simulink model "example_code_generation"  (R2024b)
settings: Solver=FixedStepDiscrete  StartTime=0.0  StopTime=40  FixedStep=0.01  RelTol=1e-3
undefined symbols (not defined in the file or in its folder): DiscIntNeverNeededParam
libraries: simulink x19, myLib x19, simulink_extras x8, mcbcontrolslib x2
settings Model: Creator=sakee  LastModifiedBy=sakee

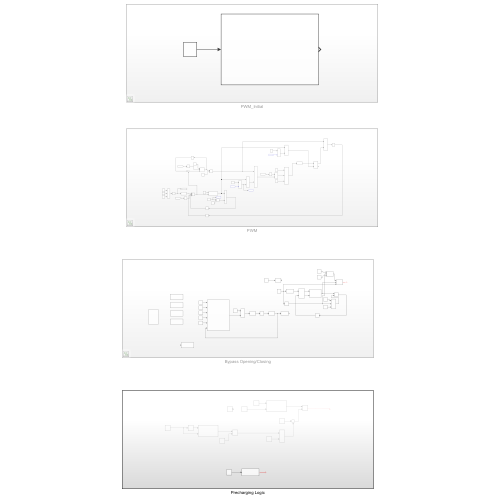
[thumbnail: Simulink's stored preview of the top-level diagram]
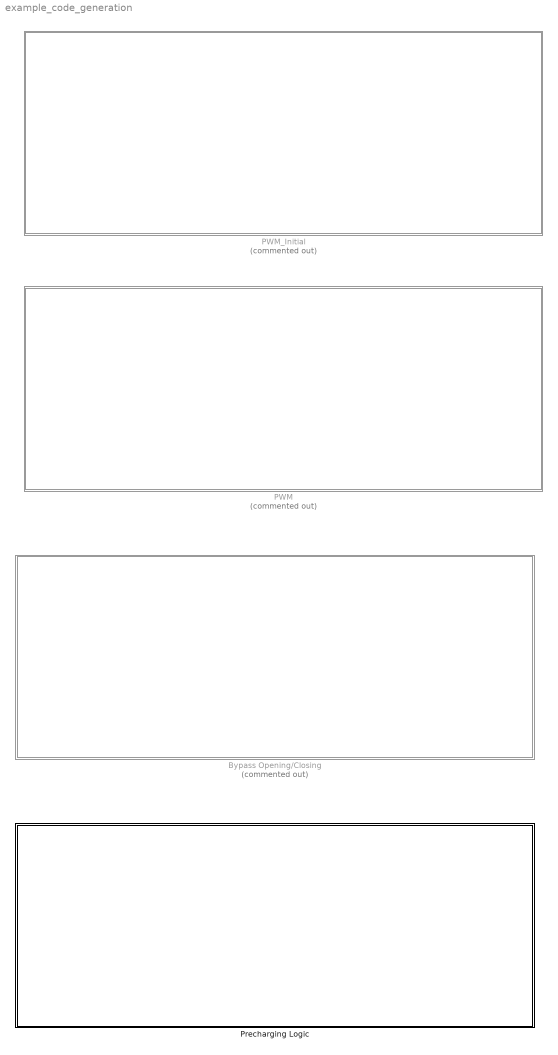
== system example_code_generation ==
  Bypass Opening/Closing : Subsystem  Commented=on
  PWM : Subsystem  Commented=on
  PWM_Initial : Subsystem  Commented=on
  Precharging Logic : Subsystem

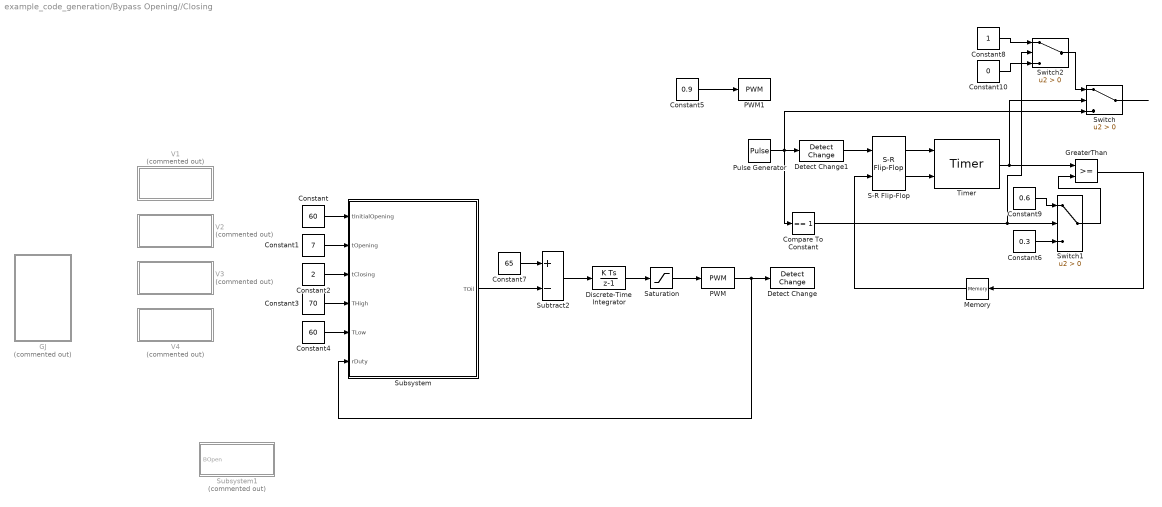
== system example_code_generation/Bypass Opening//Closing ==
  Compare To Constant : simulink/Logic and Bit Operations/Compare To Constant  relop===  const=1  OutDataTypeStr=boolean
  Constant : Constant  Value=60
  Constant1 : Constant  Value=7
  Constant10 : Constant  Value=0
  Constant2 : Constant  Value=2
  Constant3 : Constant  Value=70
  Constant4 : Constant  Value=60
  Constant5 : Constant  Value=0.9
  Constant6 : Constant  Value=0.3
  Constant7 : Constant  Value=65
  Constant8 : Constant
  Constant9 : Constant  Value=0.6
  Detect Change : simulink/Logic and Bit Operations/Detect Change  vinit=0  OutDataTypeStr=boolean
  Detect Change1 : simulink/Logic and Bit Operations/Detect Change  vinit=0  OutDataTypeStr=boolean
  Discrete-Time Integrator : DiscreteIntegrator  gainval=0.05  SampleTime=-1  LimitOutput=on  UpperSaturationLimit=1  LowerSaturationLimit=0  ICPrevOutput=DiscIntNeverNeededParam  ICPrevScaledInput=DiscIntNeverNeededParam
  GJ : Subsystem  Commented=on
  GreaterThan : RelationalOperator  OutDataTypeStr=boolean  RndMeth=Simplest  InputSameDT=off
  Memory : Memory
  PWM : simulink/Discontinuities/PWM  DisableCoverage=on  Period=0.2  InitialDelay=0  DisallowZeroDutyCycle=off  RunAtFixedTimeIntervals=on  SampleTime=0.01
  PWM1 : simulink/Discontinuities/PWM  DisableCoverage=on  Period=0.2  InitialDelay=0  DisallowZeroDutyCycle=off  RunAtFixedTimeIntervals=on  SampleTime=0.01
  Pulse Generator : DiscretePulseGenerator  PulseType=Time based  Period=1  PulseWidth=80
  S-R Flip-Flop : simulink_extras/Flip Flops/S-R Flip-Flop  initial_condition=0
  Saturation : Saturate  UpperLimit=1  LowerLimit=0
  Subsystem : Subsystem
  Subsystem1 : Subsystem  Commented=on
  Subtract2 : Sum  Inputs=+-
  Switch : Switch  Criteria=u2 > Threshold  SaturateOnIntegerOverflow=off  InputSameDT=off
  Switch1 : Switch  Criteria=u2 > Threshold  SaturateOnIntegerOverflow=off  InputSameDT=off
  Switch2 : Switch  Criteria=u2 > Threshold  SaturateOnIntegerOverflow=off  InputSameDT=off
  Timer : myLib/Timer  tSampleTime=0.01
  V1 : Subsystem  Commented=on
  V2 : Subsystem  Commented=on
  V3 : Subsystem  Commented=on
  V4 : Subsystem  Commented=on
  wires:
  Constant/1 -> Subsystem/1(tInitialOpening)
  Constant1/1 -> Subsystem/2(tOpening)
  Constant2/1 -> Subsystem/3(tClosing)
  Constant3/1 -> Subsystem/4(THigh)
  Constant4/1 -> Subsystem/5(TLow)
  Constant7/1 -> Subtract2/1
  Discrete-Time Integrator/1 -> Saturation/1
  Saturation/1 -> PWM/1
  Subtract2/1 -> Discrete-Time Integrator/1
  Subsystem/1(TOil) -> Subtract2/2
  PWM/1 -> Detect Change/1, Subsystem/6(rDuty)
  Constant5/1 -> PWM1/1
  Detect Change1/1 -> S-R Flip-Flop/1
  S-R Flip-Flop/1 -> Timer/1
  S-R Flip-Flop/2 -> Timer/2
  Timer/1 -> Switch/2, GreaterThan/1
  GreaterThan/1 -> Memory/1
  Switch1/1 -> GreaterThan/2
  Memory/1 -> S-R Flip-Flop/2
  Pulse Generator/1 -> Detect Change1/1, Switch/3, Compare To Constant/1
  Switch/1 -> ?
  Compare To Constant/1 -> Switch2/2, Switch1/2
  Constant6/1 -> Switch1/3
  Constant9/1 -> Switch1/1
  Constant8/1 -> Switch2/1
  Constant10/1 -> Switch2/3
  Switch2/1 -> Switch/1

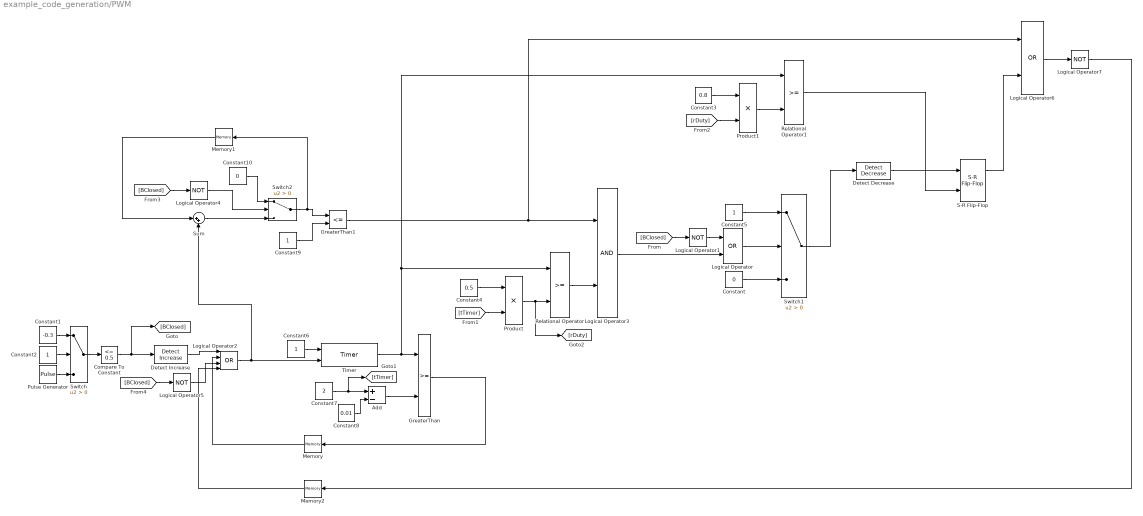
== system example_code_generation/PWM ==
  Add : Sum  Inputs=+-
  Compare To Constant : simulink/Logic and Bit Operations/Compare To Constant  relop=<=  const=0.5  OutDataTypeStr=boolean
  Constant : Constant  Value=0
  Constant1 : Constant  Value=-0.3
  Constant10 : Constant  Value=0
  Constant{2,5..6,9} (4 alike) : Constant
  Constant3 : Constant  Value=0.8
  Constant4 : Constant  Value=0.5
  Constant7 : Constant  Value=2
  Constant8 : Constant  Value=0.01
  Detect Decrease : simulink/Logic and Bit Operations/Detect Decrease  vinit=0.0  OutDataTypeStr=boolean
  Detect Increase : simulink/Logic and Bit Operations/Detect Increase  vinit=0.0  OutDataTypeStr=boolean
  GreaterThan : RelationalOperator  OutDataTypeStr=boolean  RndMeth=Simplest  InputSameDT=off
  GreaterThan1 : RelationalOperator  Operator=<=  OutDataTypeStr=boolean  RndMeth=Simplest  InputSameDT=off
  Logical Operator : Logic  Operator=OR  AllPortsSameDT=off  OutDataTypeStr=boolean
  Logical Operator{1,4..5,7} (4 alike) : Logic  Operator=NOT  AllPortsSameDT=off  OutDataTypeStr=boolean
  Logical Operator2 : Logic  Operator=OR  Inputs=4  AllPortsSameDT=off  OutDataTypeStr=boolean
  Logical Operator3 : Logic  AllPortsSameDT=off  OutDataTypeStr=boolean
  Logical Operator6 : Logic  Operator=OR  AllPortsSameDT=off  OutDataTypeStr=boolean
  Memory : Memory
  Memory1 : Memory
  Memory2 : Memory
  Product : Product
  Product1 : Product
  Pulse Generator : DiscretePulseGenerator  PulseType=Time based  Period=10  PulseWidth=50
  Relational Operator : RelationalOperator  OutDataTypeStr=boolean  RndMeth=Simplest  InputSameDT=off
  Relational Operator1 : RelationalOperator  OutDataTypeStr=boolean  RndMeth=Simplest  InputSameDT=off
  S-R Flip-Flop : simulink_extras/Flip Flops/S-R Flip-Flop  initial_condition=0
  Sum : Sum  Inputs=|++
  Switch : Switch  Criteria=u2 > Threshold  SaturateOnIntegerOverflow=off  InputSameDT=off
  Switch1 : Switch  Criteria=u2 > Threshold  SaturateOnIntegerOverflow=off  InputSameDT=off
  Switch2 : Switch  Criteria=u2 > Threshold  SaturateOnIntegerOverflow=off  InputSameDT=off
  Timer : myLib/Timer  tSampleTime=0.01
  wires:
  Product/1 -> [rDuty], Relational Operator/2
  Compare To Constant/1 -> Detect Increase/1, [BClosed]
  [BClosed] -> Logical Operator1/1
  Constant4/1 -> Product/1
  Constant/1 -> Switch1/3
  Logical Operator/1 -> Switch1/2
  Constant5/1 -> Switch1/1
  Logical Operator1/1 -> Logical Operator/1
  Constant6/1 -> Timer/1
  Pulse Generator/1 -> Switch/3
  Constant2/1 -> Switch/2
  Constant1/1 -> Switch/1
  Switch/1 -> Compare To Constant/1
  Detect Increase/1 -> Logical Operator2/1
  Constant7/1 -> [tTimer], Add/1
  Add/1 -> GreaterThan/2
  Constant8/1 -> Add/2
  GreaterThan/1 -> Memory/1
  Memory/1 -> Logical Operator2/2
  [tTimer] -> Product/2
  Logical Operator3/1 -> Logical Operator/2
  Logical Operator2/1 -> Timer/2, Sum/2
  Constant9/1 -> GreaterThan1/2
  GreaterThan1/1 -> Logical Operator6/1, Logical Operator3/1
  Switch2/1 -> Memory1/1, GreaterThan1/1
  Constant10/1 -> Switch2/1
  Sum/1 -> Switch2/3
  [BClosed] -> Logical Operator4/1
  Logical Operator4/1 -> Switch2/2
  Memory1/1 -> Sum/1
  [BClosed] -> Logical Operator5/1
  Logical Operator5/1 -> Logical Operator2/3
  Relational Operator/1 -> Logical Operator3/2
  Timer/1 -> Relational Operator1/1, Relational Operator/1, GreaterThan/1
  Constant3/1 -> Product1/1
  Product1/1 -> Relational Operator1/2
  [rDuty] -> Product1/2
  Switch1/1 -> Detect Decrease/1
  Detect Decrease/1 -> S-R Flip-Flop/1
  Relational Operator1/1 -> S-R Flip-Flop/2
  Logical Operator6/1 -> Logical Operator7/1
  Logical Operator7/1 -> Memory2/1
  Memory2/1 -> Logical Operator2/4
  S-R Flip-Flop/1 -> Logical Operator6/2

== system example_code_generation/PWM_Initial ==
  PWM : Subsystem
  Pulse Generator : DiscretePulseGenerator  PulseType=Time based  Period=10  PulseWidth=50
  wires:
  Pulse Generator/1 -> PWM/1(In1)

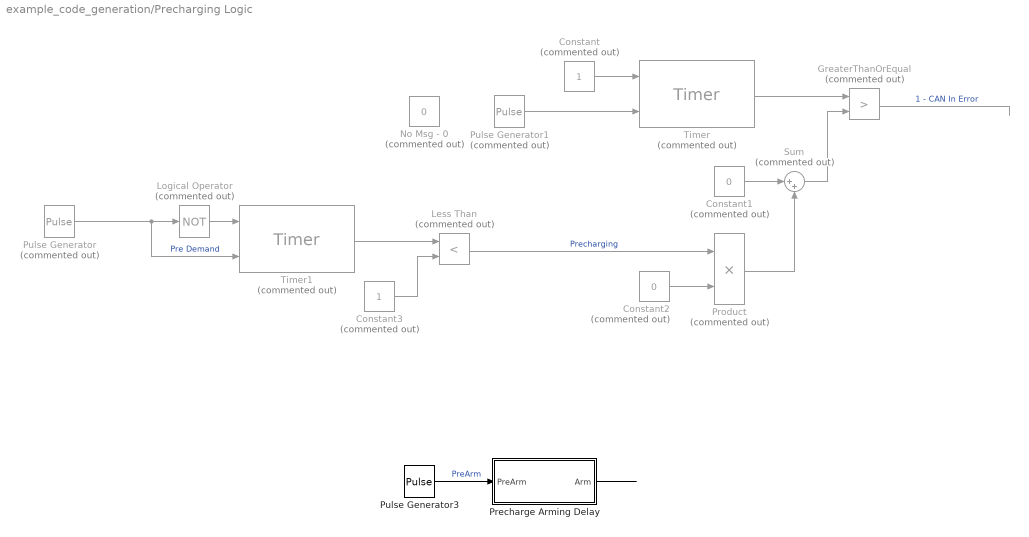
== system example_code_generation/Precharging Logic ==
  Constant : Constant  Commented=on
  Constant1 : Constant  Commented=on  Value=0
  Constant2 : Constant  Commented=on  Value=0
  Constant3 : Constant  Commented=on
  GreaterThanOrEqual : RelationalOperator  Commented=on  Operator=>  OutDataTypeStr=boolean  RndMeth=Simplest  InputSameDT=off
  Less Than : RelationalOperator  Commented=on  Operator=<  OutDataTypeStr=boolean  RndMeth=Simplest  InputSameDT=off
  Logical Operator : Logic  Commented=on  Operator=NOT  AllPortsSameDT=off  OutDataTypeStr=boolean
  No Msg - 0 : Constant  Commented=on  Value=0
  Precharge Arming Delay : Subsystem
  Product : Product  Commented=on
  Pulse Generator : DiscretePulseGenerator  Commented=on  PulseType=Time based  Period=40  PulseWidth=50
  Pulse Generator1 : DiscretePulseGenerator  Commented=on  PulseType=Time based  Period=40  PulseWidth=30
  Pulse Generator3 : DiscretePulseGenerator  PulseType=Time based  Period=10  PulseWidth=50  PhaseDelay=20
  Sum : Sum  Commented=on  Inputs=|++
  Timer : myLib/Timer  Commented=on  tSampleTime=0.01
  Timer1 : myLib/Timer  Commented=on  tSampleTime=0.01
  wires:
  Constant/1 -> Timer/1
  Timer/1 -> GreaterThanOrEqual/1
  Constant1/1 -> Sum/1
  Product/1 -> Sum/2
  Sum/1 -> GreaterThanOrEqual/2
  Constant2/1 -> Product/2
  Timer1/1 -> Less Than/1
  Constant3/1 -> Less Than/2
  Less Than/1 -> Product/1  "Precharging"
  Logical Operator/1 -> Timer1/1
  Pulse Generator/1 -> Timer1/2, Logical Operator/1  "Pre Demand"
  GreaterThanOrEqual/1 -> ?  "1 - CAN In Error"
  Pulse Generator1/1 -> Timer/2
  Pulse Generator3/1 -> Precharge Arming Delay/1(PreArm)  "PreArm"
  Precharge Arming Delay/1(Arm) -> ?

== system example_code_generation/Bypass Opening//Closing/GJ ==
  Bypass : Subsystem
  Constant4 : Constant  Value=120
  Constant5 : Constant  Value=60
  Constant7 : Constant  Value=80
  Discrete-Time Integrator : DiscreteIntegrator  gainval=0.005  SampleTime=-1  LimitOutput=on  UpperSaturationLimit=1  LowerSaturationLimit=0  ICPrevOutput=DiscIntNeverNeededParam  ICPrevScaledInput=DiscIntNeverNeededParam
  PWM : simulink/Discontinuities/PWM  DisableCoverage=on  Period=0.2  InitialDelay=0  DisallowZeroDutyCycle=off  RunAtFixedTimeIntervals=on  SampleTime=0.01
  Saturation : Saturate  UpperLimit=1  LowerLimit=0
  Subtract2 : Sum  Inputs=+-
  wires:
  Constant7/1 -> Subtract2/1
  Subtract2/1 -> Discrete-Time Integrator/1
  Constant5/1 -> Bypass/3(TClosed)
  PWM/1 -> Bypass/2(BOpen)
  Constant4/1 -> Bypass/1(TOpen)
  Saturation/1 -> PWM/1
  Discrete-Time Integrator/1 -> Saturation/1
  Bypass/1(TOil) -> Subtract2/2

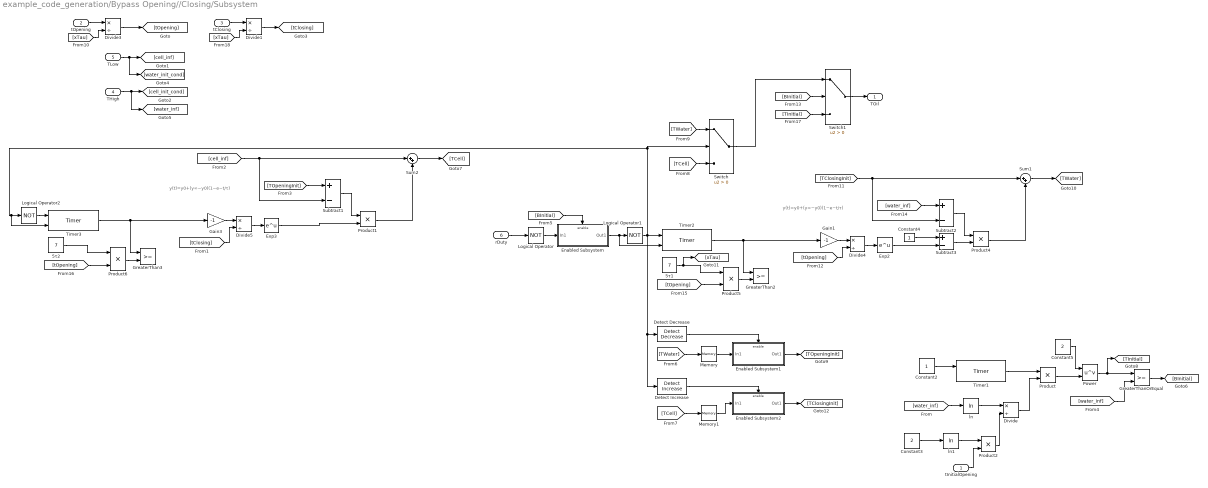
== system example_code_generation/Bypass Opening//Closing/Subsystem ==
  note: y(t)=y0​+(y∞​−y0​)(1−e−t/τ)
  note: y(t)=y0​+(y∞​−y0​)(1−e−t/τ)
  tInitialOpening : Inport
  tOpening : Inport  Port=2
  tClosing : Inport  Port=3
  THigh : Inport  Port=4
  TLow : Inport  Port=5
  rDuty : Inport  Port=6
  5τ1 : Constant  Value=7
  5τ2 : Constant  Value=7
  Constant2 : Constant
  Constant3 : Constant  Value=2
  Constant4 : Constant
  Constant5 : Constant  Value=2
  Detect Decrease : simulink/Logic and Bit Operations/Detect Decrease  vinit=0.0  OutDataTypeStr=boolean
  Detect Increase : simulink/Logic and Bit Operations/Detect Increase  vinit=0.0  OutDataTypeStr=boolean
  Divide{,1,3..5} (5 alike) : Product  Inputs=*/
  Enabled Subsystem : Subsystem  TreatAsAtomicUnit=on
  Enabled Subsystem1 : Subsystem  TreatAsAtomicUnit=on
  Enabled Subsystem2 : Subsystem  TreatAsAtomicUnit=on
  Exp2 : Math
  Exp3 : Math
  Gain1 : Gain  Gain=-1
  Gain3 : Gain  Gain=-1
  GreaterThan2 : RelationalOperator  OutDataTypeStr=boolean  RndMeth=Simplest  InputSameDT=off
  GreaterThan3 : RelationalOperator  OutDataTypeStr=boolean  RndMeth=Simplest  InputSameDT=off
  GreaterThanOrEqual : RelationalOperator  OutDataTypeStr=boolean  RndMeth=Simplest  InputSameDT=off
  Logical Operator : Logic  Operator=NOT  AllPortsSameDT=off  OutDataTypeStr=boolean
  Logical Operator1 : Logic  Operator=NOT  AllPortsSameDT=off  OutDataTypeStr=boolean
  Logical Operator2 : Logic  Operator=NOT  AllPortsSameDT=off  OutDataTypeStr=boolean
  Memory : Memory
  Memory1 : Memory
  Power : Math  Operator=pow
  Product{,1..2,4..6} (6 alike) : Product
  Subtract1 : Sum  Inputs=+-
  Subtract2 : Sum  Inputs=+-
  Subtract3 : Sum  Inputs=+-
  Sum1 : Sum  Inputs=|++
  Sum2 : Sum  Inputs=|++
  Switch : Switch  Criteria=u2 > Threshold  SaturateOnIntegerOverflow=off  InputSameDT=off
  Switch1 : Switch  Criteria=u2 > Threshold  SaturateOnIntegerOverflow=off  InputSameDT=off
  Timer1 : myLib/Timer  tSampleTime=0.01
  Timer2 : myLib/Timer  tSampleTime=0.01
  Timer3 : myLib/Timer  tSampleTime=0.01
  ln : Math  Operator=log
  ln1 : Math  Operator=log
  TOil : Outport
  wires:
  Divide3/1 -> [tOpening]
  THigh/1 -> [water_inf], [cell_init_cond]
  [xTau] -> Divide3/2
  [TWater] -> Switch/1
  TLow/1 -> [water_init_cond], [cell_inf]
  Switch/1 -> Switch1/1
  [TCell] -> Switch/3
  tOpening/1 -> Divide3/1
  Subtract3/1 -> Product4/2
  [tOpening] -> Product5/2
  Product5/1 -> GreaterThan2/2
  5τ1/1 -> Product5/1, [xTau]
  Divide4/1 -> Exp2/1
  Gain1/1 -> Divide4/1
  Constant4/1 -> Subtract3/1
  [water_inf] -> Subtract2/1
  Exp2/1 -> Subtract3/2
  [tOpening] -> Divide4/2
  Subtract2/1 -> Product4/1
  Timer2/1 -> GreaterThan2/1, Gain1/1
  Product4/1 -> Sum1/2
  [TClosingInit] -> Subtract2/2, Sum1/1
  Sum1/1 -> [TWater]
  [cell_inf] -> Sum2/1, Subtract1/2
  Product1/1 -> Sum2/2
  Timer3/1 -> Gain3/1, GreaterThan3/1
  Subtract1/1 -> Product1/1
  [tClosing] -> Divide5/2
  [TOpeningInit] -> Subtract1/1
  Gain3/1 -> Divide5/1
  Divide5/1 -> Exp3/1
  5τ2/1 -> Product6/1
  Product6/1 -> GreaterThan3/2
  [tOpening] -> Product6/2
  Sum2/1 -> [TCell]
  rDuty/1 -> Logical Operator/1
  Logical Operator/1 -> Enabled Subsystem/1(In1)
  Logical Operator1/1 -> Detect Increase/1, Detect Decrease/1, Timer3/2, Logical Operator2/1, Switch/2, Timer2/1
  Enabled Subsystem/1(Out1) -> Timer2/2, Logical Operator1/1
  Constant2/1 -> Timer1/1
  Timer1/1 -> Product/1
  [water_inf] -> ln/1
  ln/1 -> Divide/1
  Constant3/1 -> ln1/1
  ln1/1 -> Product2/1
  tInitialOpening/1 -> Product2/2
  Product2/1 -> Divide/2
  Divide/1 -> Product/2
  Product/1 -> Power/2
  Constant5/1 -> Power/1
  Power/1 -> [TInitial], GreaterThanOrEqual/1
  [water_inf] -> GreaterThanOrEqual/2
  GreaterThanOrEqual/1 -> [BInitial]
  [BInitial] -> Enabled Subsystem/Enable
  Detect Decrease/1 -> Enabled Subsystem1/Enable
  [TWater] -> Memory/1
  Memory/1 -> Enabled Subsystem1/1(In1)
  Detect Increase/1 -> Enabled Subsystem2/Enable
  [TCell] -> Memory1/1
  Memory1/1 -> Enabled Subsystem2/1(In1)
  Enabled Subsystem1/1(Out1) -> [TOpeningInit]
  Enabled Subsystem2/1(Out1) -> [TClosingInit]
  [BInitial] -> Switch1/2
  [TInitial] -> Switch1/3
  Switch1/1 -> TOil/1
  Logical Operator2/1 -> Timer3/1
  tClosing/1 -> Divide1/1
  [xTau] -> Divide1/2
  Divide1/1 -> [tClosing]
  Exp3/1 -> Product1/2

== system example_code_generation/Bypass Opening//Closing/Subsystem1 ==
  BOpen : Inport
  Hardware to Controller : Subsystem
  PWM : Subsystem
  wires:
  BOpen/1 -> PWM/1(BOpen)
  PWM/1(rDutyOut) -> Hardware to Controller/1(In1)

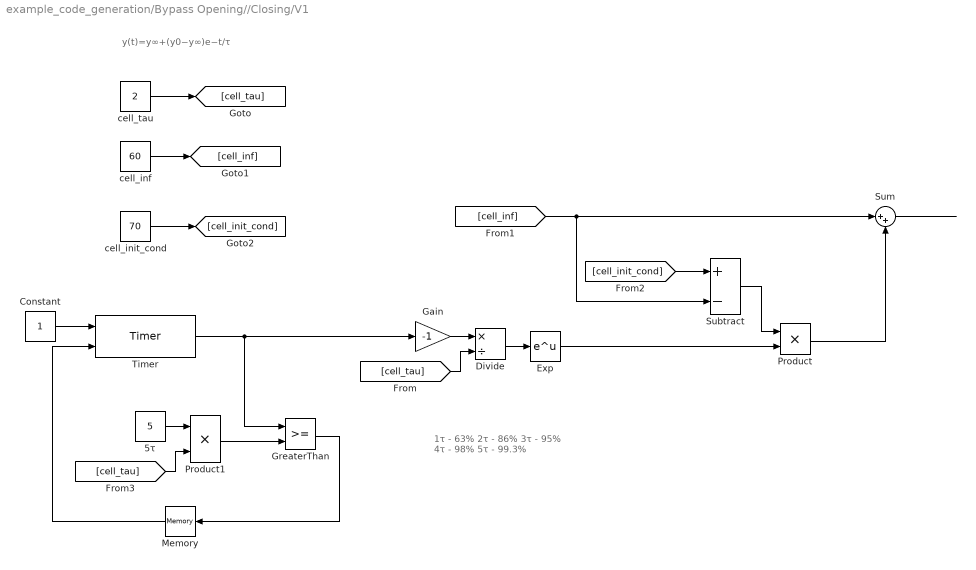
== system example_code_generation/Bypass Opening//Closing/V1 ==
  note: 1τ - 63%
      | 2τ - 86%
      | 3τ - 95%
      | 4τ - 98%
      | 5τ - 99.3%
  note: y(t)=y∞​+(y0​−y∞​)e−t/τ
  5τ : Constant  Value=5
  Constant : Constant
  Divide : Product  Inputs=*/
  Exp : Math
  Gain : Gain  Gain=-1
  GreaterThan : RelationalOperator  OutDataTypeStr=boolean  RndMeth=Simplest  InputSameDT=off
  Memory : Memory
  Product : Product
  Product1 : Product
  Subtract : Sum  Inputs=+-
  Sum : Sum  Inputs=|++
  Timer : myLib/Timer  tSampleTime=0.01
  cell_inf : Constant  Value=60
  cell_init_cond : Constant  Value=70
  cell_tau : Constant  Value=2
  wires:
  [cell_tau] -> Divide/2
  Sum/1 -> ?
  cell_inf/1 -> [cell_inf]
  cell_tau/1 -> [cell_tau]
  Product/1 -> Sum/2
  [cell_tau] -> Product1/2
  [cell_inf] -> Sum/1, Subtract/2
  [cell_init_cond] -> Subtract/1
  Timer/1 -> GreaterThan/1, Gain/1
  GreaterThan/1 -> Memory/1
  Exp/1 -> Product/2
  Subtract/1 -> Product/1
  Constant/1 -> Timer/1
  cell_init_cond/1 -> [cell_init_cond]
  Divide/1 -> Exp/1
  Gain/1 -> Divide/1
  Memory/1 -> Timer/2
  Product1/1 -> GreaterThan/2
  5τ/1 -> Product1/1

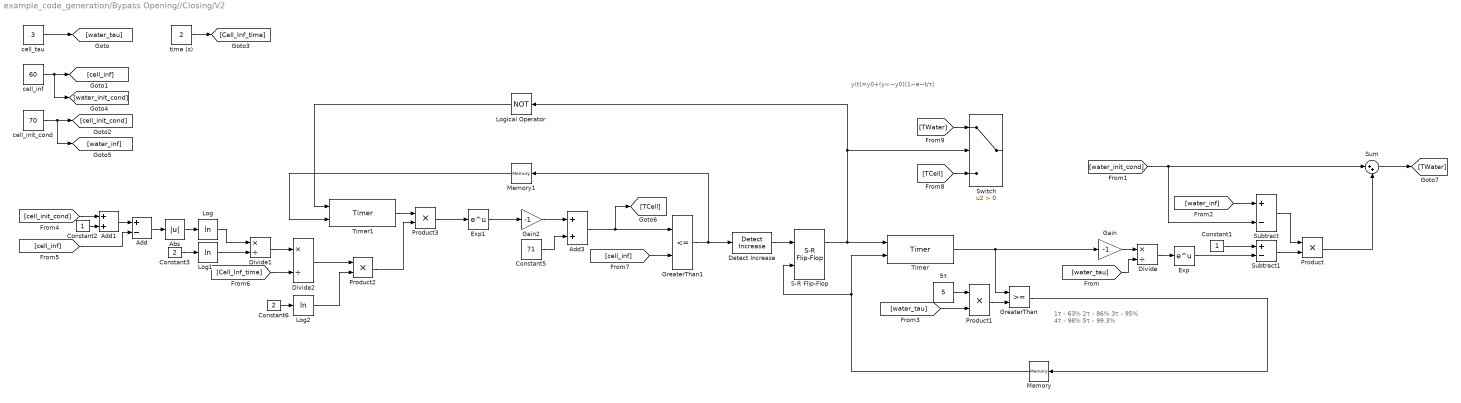
== system example_code_generation/Bypass Opening//Closing/V2 ==
  note: 1τ - 63%
      | 2τ - 86%
      | 3τ - 95%
      | 4τ - 98%
      | 5τ - 99.3%
  note: y(t)=y0​+(y∞​−y0​)(1−e−t/τ)
  5τ : Constant  Value=5
  Abs : Abs  SaturateOnIntegerOverflow=off
  Add : Sum  Inputs=+-
  Add1 : Sum
  Add3 : Sum
  Constant1 : Constant
  Constant2 : Constant
  Constant3 : Constant  Value=2
  Constant5 : Constant  Value=71
  Constant6 : Constant  Value=2
  Detect Increase : simulink/Logic and Bit Operations/Detect Increase  vinit=0.0  OutDataTypeStr=boolean
  Divide : Product  Inputs=*/
  Divide1 : Product  Inputs=*/
  Divide2 : Product  Inputs=*/
  Exp : Math
  Exp1 : Math
  Gain : Gain  Gain=-1
  Gain2 : Gain  Gain=-1
  GreaterThan : RelationalOperator  OutDataTypeStr=boolean  RndMeth=Simplest  InputSameDT=off
  GreaterThan1 : RelationalOperator  Operator=<=  OutDataTypeStr=boolean  RndMeth=Simplest  InputSameDT=off
  Log : Math  Operator=log
  Log1 : Math  Operator=log
  Log2 : Math  Operator=log
  Logical Operator : Logic  Operator=NOT  AllPortsSameDT=off  OutDataTypeStr=boolean
  Memory : Memory
  Memory1 : Memory
  Product{,1..3} (4 alike) : Product
  S-R Flip-Flop : simulink_extras/Flip Flops/S-R Flip-Flop  initial_condition=0
  Subtract : Sum  Inputs=+-
  Subtract1 : Sum  Inputs=+-
  Sum : Sum  Inputs=|++
  Switch : Switch  Criteria=u2 > Threshold  SaturateOnIntegerOverflow=off  InputSameDT=off
  Timer : myLib/Timer  tSampleTime=0.01
  Timer1 : myLib/Timer  tSampleTime=0.01
  cell_inf : Constant  Value=60
  cell_init_cond : Constant  Value=70
  cell_tau : Constant  Value=3
  time (s) : Constant  Value=2
  wires:
  Detect Increase/1 -> S-R Flip-Flop/1
  GreaterThan1/1 -> Memory1/1, Detect Increase/1
  Constant5/1 -> Add3/2
  Product2/1 -> Product3/2
  Abs/1 -> Log/1
  Sum/1 -> [TWater]
  Add/1 -> Abs/1
  [cell_init_cond] -> Add1/1
  [water_tau] -> Divide/2
  Divide2/1 -> Product2/1
  Gain2/1 -> Add3/1
  Memory1/1 -> Timer1/2
  cell_inf/1 -> [water_init_cond], [cell_inf]
  Product/1 -> Sum/2
  [water_tau] -> Product1/2
  cell_init_cond/1 -> [water_inf], [cell_init_cond]
  [water_init_cond] -> Sum/1, Subtract/2
  Divide1/1 -> Divide2/1
  Constant6/1 -> Log2/1
  time (s)/1 -> [Cell_Inf_time]
  Log2/1 -> Product2/2
  Exp1/1 -> Gain2/1
  Timer/1 -> Gain/1, GreaterThan/1
  [cell_inf] -> Add/2
  Constant2/1 -> Add1/2
  Timer1/1 -> Product3/1
  Add3/1 -> [TCell], GreaterThan1/1
  S-R Flip-Flop/1 -> Switch/2, Logical Operator/1, Timer/1
  Subtract/1 -> Product/1
  Logical Operator/1 -> Timer1/1
  Memory/1 -> S-R Flip-Flop/2, Timer/2
  Exp/1 -> Subtract1/2
  GreaterThan/1 -> Memory/1
  Subtract1/1 -> Product/2
  Constant1/1 -> Subtract1/1
  Divide/1 -> Exp/1
  Gain/1 -> Divide/1
  Log/1 -> Divide1/1
  [TWater] -> Switch/1
  Product1/1 -> GreaterThan/2
  Constant3/1 -> Log1/1
  [Cell_Inf_time] -> Divide2/2
  5τ/1 -> Product1/1
  Log1/1 -> Divide1/2
  [cell_inf] -> GreaterThan1/2
  [water_inf] -> Subtract/1
  Add1/1 -> Add/1
  cell_tau/1 -> [water_tau]
  [TCell] -> Switch/3
  Product3/1 -> Exp1/1

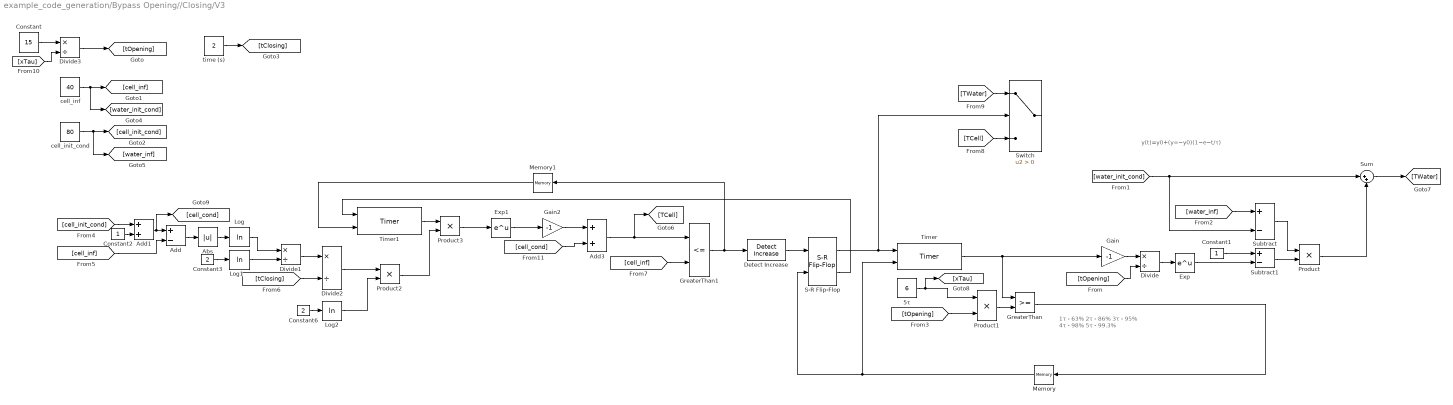
== system example_code_generation/Bypass Opening//Closing/V3 ==
  note: 1τ - 63%
      | 2τ - 86%
      | 3τ - 95%
      | 4τ - 98%
      | 5τ - 99.3%
  note: y(t)=y0​+(y∞​−y0​)(1−e−t/τ)
  5τ : Constant  Value=6
  Abs : Abs  SaturateOnIntegerOverflow=off
  Add : Sum  Inputs=+-
  Add1 : Sum
  Add3 : Sum
  Constant : Constant  Value=15
  Constant1 : Constant
  Constant2 : Constant
  Constant3 : Constant  Value=2
  Constant6 : Constant  Value=2
  Detect Increase : simulink/Logic and Bit Operations/Detect Increase  vinit=0.0  OutDataTypeStr=boolean
  Divide{,1..3} (4 alike) : Product  Inputs=*/
  Exp : Math
  Exp1 : Math
  Gain : Gain  Gain=-1
  Gain2 : Gain  Gain=-1
  GreaterThan : RelationalOperator  OutDataTypeStr=boolean  RndMeth=Simplest  InputSameDT=off
  GreaterThan1 : RelationalOperator  Operator=<=  OutDataTypeStr=boolean  RndMeth=Simplest  InputSameDT=off
  Log : Math  Operator=log
  Log1 : Math  Operator=log
  Log2 : Math  Operator=log
  Memory : Memory
  Memory1 : Memory
  Product{,1..3} (4 alike) : Product
  S-R Flip-Flop : simulink_extras/Flip Flops/S-R Flip-Flop  initial_condition=0
  Subtract : Sum  Inputs=+-
  Subtract1 : Sum  Inputs=+-
  Sum : Sum  Inputs=|++
  Switch : Switch  Criteria=u2 > Threshold  SaturateOnIntegerOverflow=off  InputSameDT=off
  Timer : myLib/Timer  tSampleTime=0.01
  Timer1 : myLib/Timer  tSampleTime=0.01
  cell_inf : Constant  Value=40
  cell_init_cond : Constant  Value=80
  time (s) : Constant  Value=2
  wires:
  Constant/1 -> Divide3/1
  Detect Increase/1 -> S-R Flip-Flop/1
  GreaterThan1/1 -> Memory1/1, Detect Increase/1
  [TWater] -> Switch/1
  [cell_cond] -> Add3/2
  Product2/1 -> Product3/2
  Abs/1 -> Log/1
  Sum/1 -> [TWater]
  Add/1 -> Abs/1
  [cell_init_cond] -> Add1/1
  [tOpening] -> Divide/2
  Divide2/1 -> Product2/1
  Gain2/1 -> Add3/1
  Memory1/1 -> Timer1/2
  cell_inf/1 -> [water_init_cond], [cell_inf]
  Product/1 -> Sum/2
  [tOpening] -> Product1/2
  cell_init_cond/1 -> [water_inf], [cell_init_cond]
  [water_init_cond] -> Sum/1, Subtract/2
  Divide1/1 -> Divide2/1
  Constant6/1 -> Log2/1
  time (s)/1 -> [tClosing]
  Log2/1 -> Product2/2
  S-R Flip-Flop/2 -> Timer1/1
  Divide3/1 -> [tOpening]
  Exp1/1 -> Gain2/1
  Timer/1 -> Gain/1, GreaterThan/1
  [cell_inf] -> Add/2
  Constant2/1 -> Add1/2
  Timer1/1 -> Product3/1
  Add3/1 -> [TCell], GreaterThan1/1
  Subtract/1 -> Product/1
  Memory/1 -> Timer/2, S-R Flip-Flop/2
  Exp/1 -> Subtract1/2
  GreaterThan/1 -> Memory/1
  Subtract1/1 -> Product/2
  Constant1/1 -> Subtract1/1
  Add1/1 -> [cell_cond], Add/1
  Product3/1 -> Exp1/1
  [TCell] -> Switch/3
  Divide/1 -> Exp/1
  Log/1 -> Divide1/1
  Product1/1 -> GreaterThan/2
  Constant3/1 -> Log1/1
  [tClosing] -> Divide2/2
  5τ/1 -> [xTau], Product1/1
  Log1/1 -> Divide1/2
  [cell_inf] -> GreaterThan1/2
  [water_inf] -> Subtract/1
  [xTau] -> Divide3/2
  S-R Flip-Flop/1 -> Switch/2, Timer/1
  Gain/1 -> Divide/1

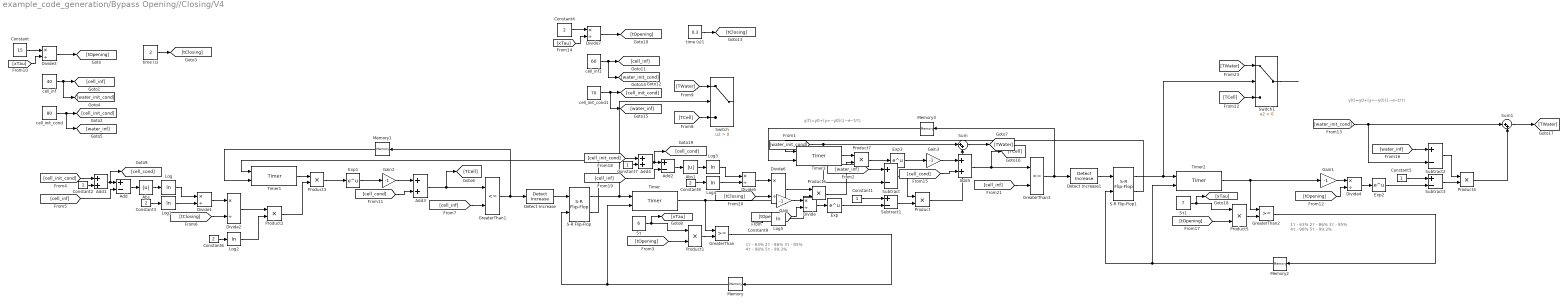
== system example_code_generation/Bypass Opening//Closing/V4 ==
  note: y(t)=y0​+(y∞​−y0​)(1−e−t/τ)
  note: 1τ - 63%
      | 2τ - 86%
      | 3τ - 95%
      | 4τ - 98%
      | 5τ - 99.3%
  note: 1τ - 63%
      | 2τ - 86%
      | 3τ - 95%
      | 4τ - 98%
      | 5τ - 99.3%
  note: y(t)=y0​+(y∞​−y0​)(1−e−t/τ)
  5τ : Constant  Value=6
  5τ1 : Constant  Value=7
  Abs : Abs  SaturateOnIntegerOverflow=off
  Abs1 : Abs  SaturateOnIntegerOverflow=off
  Add : Sum  Inputs=+-
  Add{1,3..5} (4 alike) : Sum
  Add2 : Sum  Inputs=+-
  Constant : Constant  Value=15
  Constant{1..2,5,7} (4 alike) : Constant
  Constant{3..4,6,8..9} (5 alike) : Constant  Value=2
  Detect Increase : simulink/Logic and Bit Operations/Detect Increase  vinit=0.0  OutDataTypeStr=boolean
  Detect Increase1 : simulink/Logic and Bit Operations/Detect Increase  vinit=0.0  OutDataTypeStr=boolean
  Divide{,1..7} (8 alike) : Product  Inputs=*/
  Exp{,1..3} (4 alike) : Math
  Gain{,1..3} (4 alike) : Gain  Gain=-1
  GreaterThan : RelationalOperator  OutDataTypeStr=boolean  RndMeth=Simplest  InputSameDT=off
  GreaterThan1 : RelationalOperator  Operator=<=  OutDataTypeStr=boolean  RndMeth=Simplest  InputSameDT=off
  GreaterThan2 : RelationalOperator  OutDataTypeStr=boolean  RndMeth=Simplest  InputSameDT=off
  GreaterThan3 : RelationalOperator  Operator=<=  OutDataTypeStr=boolean  RndMeth=Simplest  InputSameDT=off
  Log{,1..5} (6 alike) : Math  Operator=log
  Memory{,1..3} (4 alike) : Memory
  Product{,1..7} (8 alike) : Product
  S-R Flip-Flop : simulink_extras/Flip Flops/S-R Flip-Flop  initial_condition=0
  S-R Flip-Flop1 : simulink_extras/Flip Flops/S-R Flip-Flop  initial_condition=0
  Subtract{,1..3} (4 alike) : Sum  Inputs=+-
  Sum : Sum  Inputs=|++
  Sum1 : Sum  Inputs=|++
  Switch : Switch  Criteria=u2 > Threshold  SaturateOnIntegerOverflow=off  InputSameDT=off
  Switch1 : Switch  Criteria=u2 > Threshold  SaturateOnIntegerOverflow=off  InputSameDT=off
  Timer{,1..3} (4 alike) : myLib/Timer  tSampleTime=0.01
  cell_inf : Constant  Value=40
  cell_inf1 : Constant  Value=60
  cell_init_cond : Constant  Value=80
  cell_init_cond1 : Constant  Value=70
  time (s) : Constant  Value=2
  time (s)1 : Constant  Value=0.3
  wires:
  Gain/1 -> Divide/1
  S-R Flip-Flop/1 -> Timer/1, Switch/2
  [xTau] -> Divide3/2
  [water_inf] -> Subtract/1
  [cell_inf] -> GreaterThan1/2
  Log1/1 -> Divide1/2
  5τ/1 -> Product1/1, [xTau]
  [tClosing] -> Divide2/2
  Constant3/1 -> Log1/1
  Product1/1 -> GreaterThan/2
  Log/1 -> Divide1/1
  Divide/1 -> Exp/1
  [TCell] -> Switch/3
  Product3/1 -> Exp1/1
  Add1/1 -> Add/1, [cell_cond]
  Constant1/1 -> Subtract1/1
  Subtract1/1 -> Product/2
  GreaterThan/1 -> Memory/1
  Exp/1 -> Subtract1/2
  Memory/1 -> S-R Flip-Flop/2, Timer/2
  Subtract/1 -> Product/1
  Add3/1 -> GreaterThan1/1, [TCell]
  Timer1/1 -> Product3/1
  Constant2/1 -> Add1/2
  [cell_inf] -> Add/2
  Timer/1 -> GreaterThan/1, Gain/1
  Exp1/1 -> Gain2/1
  Divide3/1 -> [tOpening]
  S-R Flip-Flop/2 -> Timer1/1
  Log2/1 -> Product2/2
  time (s)/1 -> [tClosing]
  Constant6/1 -> Log2/1
  Divide1/1 -> Divide2/1
  [water_init_cond] -> Subtract/2, Sum/1
  cell_init_cond/1 -> [cell_init_cond], [water_inf]
  [tOpening] -> Product1/2
  Product/1 -> Sum/2
  cell_inf/1 -> [cell_inf], [water_init_cond]
  Memory1/1 -> Timer1/2
  Gain2/1 -> Add3/1
  Divide2/1 -> Product2/1
  [tOpening] -> Divide/2
  [cell_init_cond] -> Add1/1
  Add/1 -> Abs/1
  Sum/1 -> [TWater]
  Abs/1 -> Log/1
  Product2/1 -> Product3/2
  [cell_cond] -> Add3/2
  [TWater] -> Switch/1
  GreaterThan1/1 -> Detect Increase/1, Memory1/1
  Detect Increase/1 -> S-R Flip-Flop/1
  Constant/1 -> Divide3/1
  S-R Flip-Flop1/1 -> Switch1/2, Timer2/1
  Divide7/1 -> [tOpening]
  Exp3/1 -> Gain3/1
  Detect Increase1/1 -> S-R Flip-Flop1/1
  Sum1/1 -> [TWater]
  [water_init_cond] -> Sum1/1, Subtract2/2
  Product4/1 -> Sum1/2
  Timer2/1 -> Gain1/1, GreaterThan2/1
  cell_init_cond1/1 -> [water_inf], [cell_init_cond]
  Subtract2/1 -> Product4/1
  [tOpening] -> Divide4/2
  time (s)1/1 -> [tClosing]
  [xTau] -> Divide7/2
  Log5/1 -> Product6/2
  Log3/1 -> Divide5/1
  [TWater] -> Switch1/1
  Gain3/1 -> Add5/1
  Product6/1 -> Product7/2
  Divide5/1 -> Divide6/1
  Constant8/1 -> Log4/1
  Exp2/1 -> Subtract3/2
  [tClosing] -> Divide6/2
  [water_inf] -> Subtract2/1
  Constant5/1 -> Subtract3/1
  cell_inf1/1 -> [water_init_cond], [cell_inf]
  Gain1/1 -> Divide4/1
  Abs1/1 -> Log3/1
  Divide6/1 -> Product6/1
  Switch1/1 -> ?
  Timer3/1 -> Product7/1
  [cell_cond] -> Add5/2
  Divide4/1 -> Exp2/1
  Add4/1 -> [cell_cond], Add2/1
  [cell_inf] -> GreaterThan3/2
  5τ1/1 -> [xTau], Product5/1
  Add5/1 -> [TCell], GreaterThan3/1
  Constant9/1 -> Log5/1
  Log4/1 -> Divide5/2
  GreaterThan3/1 -> Memory3/1, Detect Increase1/1
  S-R Flip-Flop1/2 -> Timer3/1
  Memory3/1 -> Timer3/2
  Product5/1 -> GreaterThan2/2
  [TCell] -> Switch1/3
  Add2/1 -> Abs1/1
  [tOpening] -> Product5/2
  Subtract3/1 -> Product4/2
  Constant7/1 -> Add4/2
  Memory2/1 -> Timer2/2, S-R Flip-Flop1/2
  [cell_init_cond] -> Add4/1
  Constant4/1 -> Divide7/1
  GreaterThan2/1 -> Memory2/1
  Product7/1 -> Exp3/1
  [cell_inf] -> Add2/2

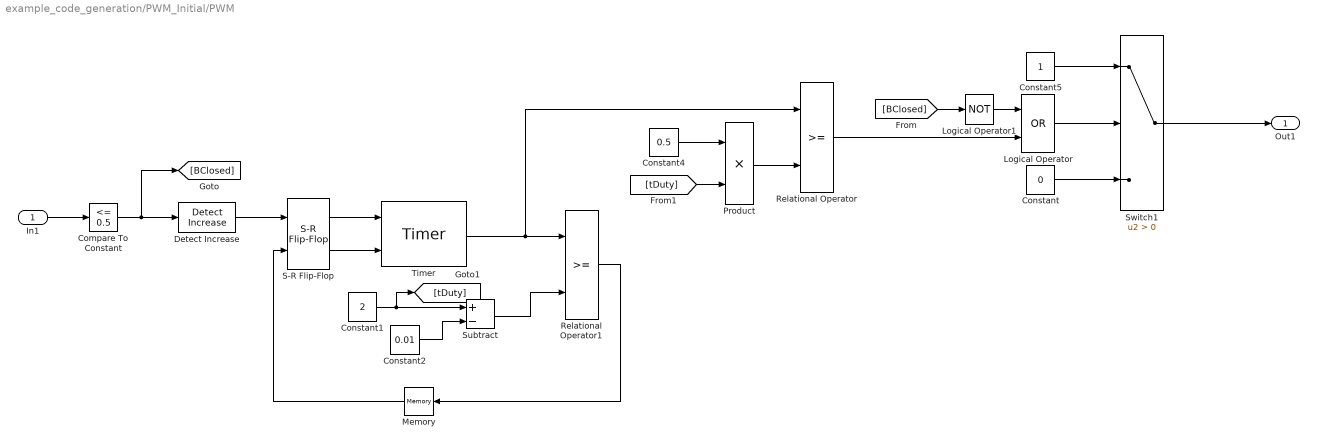
== system example_code_generation/PWM_Initial/PWM ==
  In1 : Inport
  Compare To Constant : simulink/Logic and Bit Operations/Compare To Constant  relop=<=  const=0.5  OutDataTypeStr=boolean
  Constant : Constant  Value=0
  Constant1 : Constant  Value=2
  Constant2 : Constant  Value=0.01
  Constant4 : Constant  Value=0.5
  Constant5 : Constant
  Detect Increase : simulink/Logic and Bit Operations/Detect Increase  vinit=0.0  OutDataTypeStr=boolean
  Logical Operator : Logic  Operator=OR  AllPortsSameDT=off  OutDataTypeStr=boolean
  Logical Operator1 : Logic  Operator=NOT  AllPortsSameDT=off  OutDataTypeStr=boolean
  Memory : Memory
  Product : Product
  Relational Operator : RelationalOperator  OutDataTypeStr=boolean  RndMeth=Simplest  InputSameDT=off
  Relational Operator1 : RelationalOperator  OutDataTypeStr=boolean  RndMeth=Simplest  InputSameDT=off
  S-R Flip-Flop : simulink_extras/Flip Flops/S-R Flip-Flop  initial_condition=0
  Subtract : Sum  Inputs=+-
  Switch1 : Switch  Criteria=u2 > Threshold  SaturateOnIntegerOverflow=off  InputSameDT=off
  Timer : myLib/Timer  tSampleTime=0.01
  Out1 : Outport
  wires:
  Compare To Constant/1 -> [BClosed], Detect Increase/1
  Constant4/1 -> Product/1
  Product/1 -> Relational Operator/2
  Detect Increase/1 -> S-R Flip-Flop/1
  Switch1/1 -> Out1/1
  Constant5/1 -> Switch1/1
  Logical Operator/1 -> Switch1/2
  Relational Operator/1 -> Logical Operator/2
  Constant/1 -> Switch1/3
  Logical Operator1/1 -> Logical Operator/1
  [BClosed] -> Logical Operator1/1
  In1/1 -> Compare To Constant/1
  S-R Flip-Flop/1 -> Timer/1
  S-R Flip-Flop/2 -> Timer/2
  Timer/1 -> Relational Operator/1, Relational Operator1/1
  Subtract/1 -> Relational Operator1/2
  Constant1/1 -> [tDuty], Subtract/1
  Constant2/1 -> Subtract/2
  Relational Operator1/1 -> Memory/1
  Memory/1 -> S-R Flip-Flop/2
  [tDuty] -> Product/2

== system example_code_generation/Precharging Logic/Precharge Arming Delay ==
  PreArm : Inport
  Constant4 : Constant
  Constant5 : Constant  Value=0
  Constant6 : Constant  Value=0
  GreaterThanOrEqual1 : RelationalOperator  Operator=>  OutDataTypeStr=boolean  RndMeth=Simplest  InputSameDT=off
  Logical Operator1 : Logic  Operator=NOT  AllPortsSameDT=off  OutDataTypeStr=boolean
  Product1 : Product
  Pulse Generator2 : DiscretePulseGenerator  PulseType=Time based  Period=40  PulseWidth=80
  Sum1 : Sum  Inputs=|++
  Timer2 : myLib/Timer  tSampleTime=0.01
  Arm : Outport
  wires:
  Timer2/1 -> GreaterThanOrEqual1/1
  Constant5/1 -> Sum1/1
  Constant6/1 -> Product1/2
  Pulse Generator2/1 -> Product1/1  "Pre Charging"
  Sum1/1 -> GreaterThanOrEqual1/2
  Constant4/1 -> Timer2/1
  Product1/1 -> Sum1/2
  GreaterThanOrEqual1/1 -> Arm/1
  Logical Operator1/1 -> Timer2/2
  PreArm/1 -> Logical Operator1/1

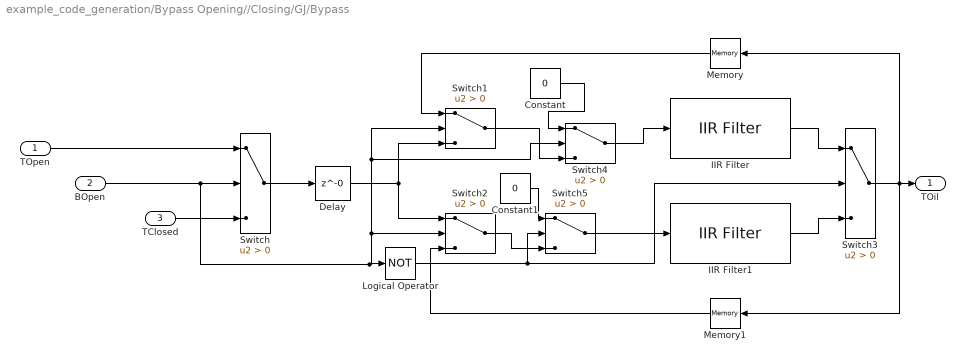
== system example_code_generation/Bypass Opening//Closing/GJ/Bypass ==
  TOpen : Inport
  BOpen : Inport  Port=2
  TClosed : Inport  Port=3
  Constant : Constant  Value=0
  Constant1 : Constant  Value=0
  Delay : Delay  DelayLength=0
  IIR Filter : mcbcontrolslib/IIR Filter  VariantControl=Low Pass Filter  VariantSelect=Low-pass  FilterConstantInputType=Specify via dialog  Filter_constant=0.9  advancedSettings=off  Ts=50e-6  cutOff_freq=28647.8898
      settings: LibrarySourceBlock=mcbhdllib/Signal Management/IIR Filter
  IIR Filter1 : mcbcontrolslib/IIR Filter  VariantControl=Low Pass Filter  VariantSelect=Low-pass  FilterConstantInputType=Specify via dialog  Filter_constant=0.9  advancedSettings=off  Ts=50e-6  cutOff_freq=28647.8898
      settings: LibrarySourceBlock=mcbhdllib/Signal Management/IIR Filter
  Logical Operator : Logic  Operator=NOT  AllPortsSameDT=off  OutDataTypeStr=boolean
  Memory : Memory
  Memory1 : Memory
  Switch{,1..5} (6 alike) : Switch  Criteria=u2 > Threshold  SaturateOnIntegerOverflow=off  InputSameDT=off
  TOil : Outport
  wires:
  TOpen/1 -> Switch/1
  BOpen/1 -> Logical Operator/1, Switch2/2, Switch4/2, Switch1/2, Switch/2
  TClosed/1 -> Switch/3
  Switch/1 -> Delay/1
  Delay/1 -> Switch2/1, Switch1/3
  Switch3/1 -> Memory1/1, Memory/1, TOil/1
  Memory/1 -> Switch1/1
  Memory1/1 -> Switch2/3
  IIR Filter/1 -> Switch3/1
  IIR Filter1/1 -> Switch3/3
  Logical Operator/1 -> Switch5/2, Switch3/2
  Constant/1 -> Switch4/1
  Switch1/1 -> Switch4/3
  Switch4/1 -> IIR Filter/1
  Constant1/1 -> Switch5/1
  Switch2/1 -> Switch5/3
  Switch5/1 -> IIR Filter1/1

== system example_code_generation/Bypass Opening//Closing/Subsystem/Enabled Subsystem ==
  In1 : Inport
  Enable : EnablePort
  Out1 : Outport
  wires:
  In1/1 -> Out1/1

== system example_code_generation/Bypass Opening//Closing/Subsystem/Enabled Subsystem1 ==
  In1 : Inport
  Enable : EnablePort
  Out1 : Outport
  wires:
  In1/1 -> Out1/1

== system example_code_generation/Bypass Opening//Closing/Subsystem/Enabled Subsystem2 ==
  In1 : Inport
  Enable : EnablePort
  Out1 : Outport
  wires:
  In1/1 -> Out1/1

== system example_code_generation/Bypass Opening//Closing/Subsystem1/Hardware to Controller ==
  In1 : Inport
  Out1 : Outport
  wires:
  In1/1 -> Out1/1

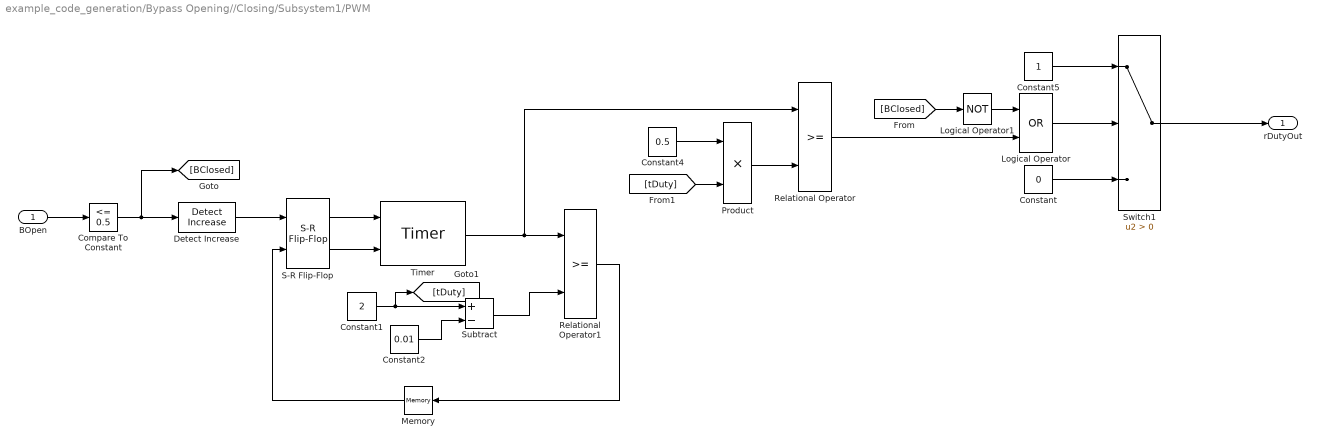
== system example_code_generation/Bypass Opening//Closing/Subsystem1/PWM ==
  BOpen : Inport
  Compare To Constant : simulink/Logic and Bit Operations/Compare To Constant  relop=<=  const=0.5  OutDataTypeStr=boolean
  Constant : Constant  Value=0
  Constant1 : Constant  Value=2
  Constant2 : Constant  Value=0.01
  Constant4 : Constant  Value=0.5
  Constant5 : Constant
  Detect Increase : simulink/Logic and Bit Operations/Detect Increase  vinit=0.0  OutDataTypeStr=boolean
  Logical Operator : Logic  Operator=OR  AllPortsSameDT=off  OutDataTypeStr=boolean
  Logical Operator1 : Logic  Operator=NOT  AllPortsSameDT=off  OutDataTypeStr=boolean
  Memory : Memory
  Product : Product
  Relational Operator : RelationalOperator  OutDataTypeStr=boolean  RndMeth=Simplest  InputSameDT=off
  Relational Operator1 : RelationalOperator  OutDataTypeStr=boolean  RndMeth=Simplest  InputSameDT=off
  S-R Flip-Flop : simulink_extras/Flip Flops/S-R Flip-Flop  initial_condition=0
  Subtract : Sum  Inputs=+-
  Switch1 : Switch  Criteria=u2 > Threshold  SaturateOnIntegerOverflow=off  InputSameDT=off
  Timer : myLib/Timer  tSampleTime=0.01
  rDutyOut : Outport
  wires:
  Compare To Constant/1 -> [BClosed], Detect Increase/1
  Constant4/1 -> Product/1
  Product/1 -> Relational Operator/2
  Detect Increase/1 -> S-R Flip-Flop/1
  Switch1/1 -> rDutyOut/1
  Constant5/1 -> Switch1/1
  Logical Operator/1 -> Switch1/2
  Relational Operator/1 -> Logical Operator/2
  Constant/1 -> Switch1/3
  Logical Operator1/1 -> Logical Operator/1
  [BClosed] -> Logical Operator1/1
  BOpen/1 -> Compare To Constant/1
  S-R Flip-Flop/1 -> Timer/1
  S-R Flip-Flop/2 -> Timer/2
  Timer/1 -> Relational Operator/1, Relational Operator1/1
  Subtract/1 -> Relational Operator1/2
  Constant1/1 -> [tDuty], Subtract/1
  Constant2/1 -> Subtract/2
  Relational Operator1/1 -> Memory/1
  Memory/1 -> S-R Flip-Flop/2
  [tDuty] -> Product/2
